simulink library "Blocks_Library"  (R2022b)
settings: Solver=VariableStepAuto  StartTime=0.0  StopTime=10.0  RelTol=1e-3
undefined symbols (not defined in the file): dataName, enumName, enumValue, raptor_xcp_function
libraries: Raptor_lib x13, $bdroot x2, simulink x1, simulink_extras x1
settings Model: Creator=jackh  LastModifiedBy=jackh

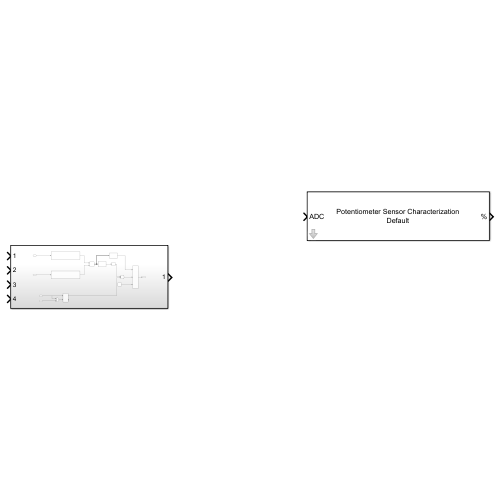
[thumbnail: Simulink's stored preview of the top-level diagram]
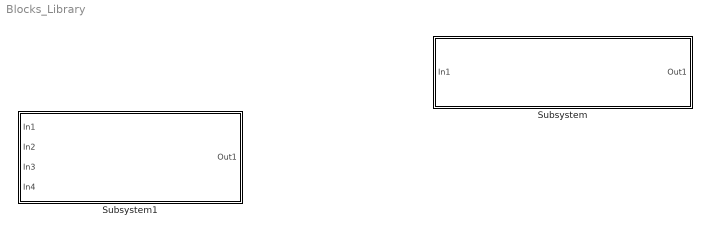
== system Blocks_Library ==
  Subsystem : Subsystem  mask{nam=Default}
      mask prompts: nam "Name"
      mask Display:
      | n = get_param(gcb, 'nam');
      | disp(['Potentiometer Sensor Characterization\n' n]);
      | port_label('input', 1, 'ADC');
      | port_label('output', 1, '%');
  Subsystem1 : Subsystem

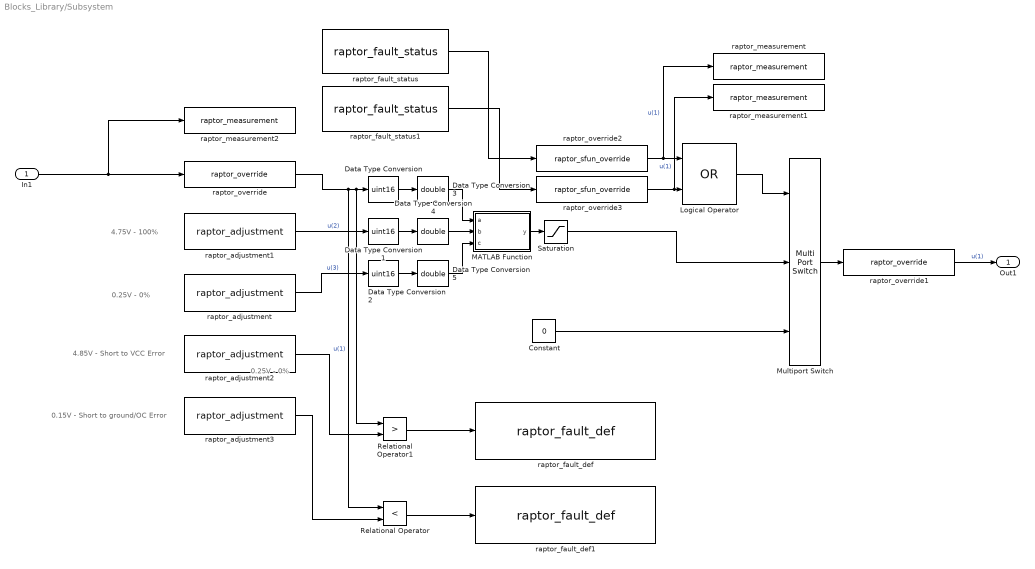
== system Blocks_Library/Subsystem ==
  note: 0.25V - 0%
  note: 4.75V - 100%
  note: 0.25V - 0%
  note: 4.85V - Short to VCC Error
  note: 0.15V - Short to ground/OC Error
  In1 : Inport
  Constant : Constant  Value=0
  Data Type Conversion : DataTypeConversion  OutDataTypeStr=uint16  SaturateOnIntegerOverflow=off  RndMeth=Floor
  Data Type Conversion1 : DataTypeConversion  OutDataTypeStr=uint16  SaturateOnIntegerOverflow=off  RndMeth=Floor
  Data Type Conversion2 : DataTypeConversion  OutDataTypeStr=uint16  SaturateOnIntegerOverflow=off  RndMeth=Floor
  Data Type Conversion3 : DataTypeConversion  OutDataTypeStr=double  SaturateOnIntegerOverflow=off  RndMeth=Floor
  Data Type Conversion4 : DataTypeConversion  OutDataTypeStr=double  SaturateOnIntegerOverflow=off  RndMeth=Floor
  Data Type Conversion5 : DataTypeConversion  OutDataTypeStr=double  SaturateOnIntegerOverflow=off  RndMeth=Floor
  Logical Operator : Logic  Operator=OR  IconShape=distinctive  AllPortsSameDT=off  OutDataTypeStr=boolean
  MATLAB Function : MATLAB Function  TreatAsAtomicUnit=on
  Multiport Switch : MultiPortSwitch  DataPortOrder=Zero-based contiguous  Inputs=2  zeroidx=on  SaturateOnIntegerOverflow=off  InputSameDT=off
  Relational Operator : RelationalOperator  Operator=<  OutDataTypeStr=boolean  RndMeth=Simplest  InputSameDT=off
  Relational Operator1 : RelationalOperator  Operator=>  OutDataTypeStr=boolean  RndMeth=Simplest  InputSameDT=off
  Saturation : Saturate  UpperLimit=100  LowerLimit=0
  raptor_adjustment : Raptor_lib/Data Storage/raptor_adjustment  paramName=[nam '_ADCLoPT']  nameSource=Parameter  initValue=205  dataType=double  storage=Constant (FLASH)  calDispType=Number  calEnum={'False', 'True'}  calGain=1.0  calOffset=0.0  calMax=inf  calMin=-inf  calFormat='-1'  calUnit='ADC'  calHelp="\"ADC Low Point\""  calAccess=1  calFunction=raptor_xcp_function(gcb)  calDispHeaders=off  calColHeaders={'Col1' 'Col2' 'Col3'}  calRowHeaders={'Row1' 'Row2' 'Row3'}
      settings: SourceProductName=Raptor
  raptor_adjustment1 : Raptor_lib/Data Storage/raptor_adjustment  paramName=[nam '_ADCHiPT']  nameSource=Parameter  initValue=3890  dataType=double  storage=Constant (FLASH)  calDispType=Number  calEnum={'False', 'True'}  calGain=1.0  calOffset=0.0  calMax=inf  calMin=-inf  calFormat='-1'  calUnit='ADC'  calHelp="\"ADC High Point\""  calAccess=1  calFunction=raptor_xcp_function(gcb)  calDispHeaders=off  calColHeaders={'Col1' 'Col2' 'Col3'}  calRowHeaders={'Row1' 'Row2' 'Row3'}
      settings: SourceProductName=Raptor
  raptor_adjustment2 : Raptor_lib/Data Storage/raptor_adjustment  paramName=[nam '_InputHighThresh']  nameSource=Parameter  initValue=3972  dataType=double  storage=Constant (FLASH)  calDispType=Number  calEnum={'False', 'True'}  calGain=1.0  calOffset=0.0  calMax=inf  calMin=-inf  calFormat='-1'  calUnit='ADC'  calHelp="\"Input out of range high point threshold\""  calAccess=1  calFunction=raptor_xcp_function(gcb)  calDispHeaders=off  calColHeaders={'Col1' 'Col2' 'Col3'}  calRowHeaders={'Row1' 'Row2' 'Row3'}
      settings: SourceProductName=Raptor
  raptor_adjustment3 : Raptor_lib/Data Storage/raptor_adjustment  paramName=[nam '_InputLowThresh']  nameSource=Parameter  initValue=123  dataType=double  storage=Constant (FLASH)  calDispType=Number  calEnum={'False', 'True'}  calGain=1.0  calOffset=0.0  calMax=inf  calMin=-inf  calFormat='-1'  calUnit='ADC'  calHelp="\"Input out of range low point threshold\""  calAccess=1  calFunction=raptor_xcp_function(gcb)  calDispHeaders=off  calColHeaders={'Col1' 'Col2' 'Col3'}  calRowHeaders={'Row1' 'Row2' 'Row3'}
      settings: SourceProductName=Raptor
  raptor_fault_def : Raptor_lib/Faults/raptor_fault_def  faultName=[nam '_InputHi']  persist=off  sticky=off  emisRelated=off  singleTrip=off  clearMethod=Standard  xLimit=25  yLimit=50  calEnable=on  addDisable=off  calAccess=4  calFunction='System | FaultManager'
      settings: SourceProductName=Raptor
  raptor_fault_def1 : Raptor_lib/Faults/raptor_fault_def  faultName=[nam '_InputLow']  persist=off  sticky=off  emisRelated=off  singleTrip=off  clearMethod=Standard  xLimit=25  yLimit=50  calEnable=on  addDisable=off  calAccess=4  calFunction='System | FaultManager'
      settings: SourceProductName=Raptor
  raptor_fault_status : Raptor_lib/Faults/raptor_fault_status  faultSource=Parameter  faultName=[nam '_InputHi']  notOccurred=off  suspected=off  active=on  occurred=off  failedThisDC=off  testCmpltThisDC=off  failing=off  pending=on  confirmed=on  mil=on  permanent=off  ready=on  prevConfirmed=off  failedSinceClear=off  failedLastDC=off  prevMil=off
      settings: SourceProductName=Raptor
  raptor_fault_status1 : Raptor_lib/Faults/raptor_fault_status  faultSource=Parameter  faultName=[nam '_InputLow']  notOccurred=off  suspected=off  active=on  occurred=off  failedThisDC=off  testCmpltThisDC=off  failing=off  pending=on  confirmed=on  mil=on  permanent=off  ready=on  prevConfirmed=off  failedSinceClear=off  failedLastDC=off  prevMil=off
      settings: SourceProductName=Raptor
  raptor_measurement : Raptor_lib/Data Storage/raptor_measurement  paramName=[nam 'HighProbe']  nameSource=Parameter  calDispType=Number  calEnum={'False', 'True'}  calGain=1.0  calOffset=0.0  calMax=inf  calMin=-inf  calFormat='-1'  calUnit=''  calHelp=''  calAccess=1  calFunction=raptor_xcp_function(gcb)  calVisible=on
      settings: SourceProductName=Raptor
  raptor_measurement1 : Raptor_lib/Data Storage/raptor_measurement  paramName=[nam 'LowProbe']  nameSource=Parameter  calDispType=Number  calEnum={'False', 'True'}  calGain=1.0  calOffset=0.0  calMax=inf  calMin=-inf  calFormat='-1'  calUnit=''  calHelp=''  calAccess=1  calFunction=raptor_xcp_function(gcb)  calVisible=on
      settings: SourceProductName=Raptor
  raptor_measurement2 : Raptor_lib/Data Storage/raptor_measurement  paramName=[nam '_ADC_Raw']  nameSource=Parameter  calDispType=Number  calEnum={'False', 'True'}  calGain=1.0  calOffset=0.0  calMax=inf  calMin=-inf  calFormat='-1'  calUnit=''  calHelp=''  calAccess=1  calFunction=raptor_xcp_function(gcb)  calVisible=on
      settings: SourceProductName=Raptor
  raptor_override : Raptor_lib/Data Storage/raptor_override  paramName=[nam '_ADC']  nameSource=Parameter  measurement=Output  calDispType=Number  calEnum={'False', 'True'}  calGain=1.0  calOffset=0.0  calMax=inf  calMin=-inf  calFormat='-1'  calUnit=''  calHelp=''  calAccess=1  calFunction="[raptor_xcp_function(gcb) '|'  'Override']"
      settings: SourceProductName=Raptor
  raptor_override1 : Raptor_lib/Data Storage/raptor_override  paramName=nam  nameSource=Parameter  measurement=Output  calDispType=Number  calEnum={'False', 'True'}  calGain=1.0  calOffset=0.0  calMax=inf  calMin=-inf  calFormat='-1'  calUnit=''  calHelp=''  calAccess=1  calFunction="[raptor_xcp_function(gcb) '|'  'Override']"
      settings: SourceProductName=Raptor
  raptor_override2 : S-Function  FunctionName=raptor_sfun_override  Parameters=char({dataName,''}), uint8(calDispType), char(enumName), int32(enumValue), double(calGain), double(calOffset), double(calMax), double(calMin), char(calUnit), char(calHelp), char(calFormat), char(calFunction), char(calAccess), uint8(measurement)  SFunctionDeploymentMode=off  EnableBusSupport=off  mask(Override){paramName=[nam '_InputHi_Override'], nameSource=Parameter, measurement=Output, calDispType=Number, calEnum={'False', 'True'}, calGain=1.0, calOffset=0.0, calMax=inf, calMin=-inf, calFormat='-1', calUnit='', calHelp='', calAccess=1, calFunction=[raptor_xcp_function(gcb) '|'  'Override']}
      mask prompts: paramName "Name:"; nameSource "Name Source:"; measurement "Add Measurement to:"; calDispType "Display as:"; calEnum "Enumeration Definition:"; calGain "Gain:"; calOffset "Offset:"; calMax "Max:"; calMin "Min:"; calFormat "Display Decimal Format:"; calUnit "Unit Text:"; calHelp "Help Text:"; calAccess "Access Level"; calFunction "Function"
      mask help: This block is used to modify the value on a wire as needed from the calibration tool.
      mask init:
      | raptor_sfun_override_maskInit;
      settings: MoveFcn=raptor_icon_redraw(gcb);
      mask Help: eval('raptor_help(''raptor_override'');')
      mask TypeOptions nameSource: Parameter | Input Wire | Output Wire
      mask Callback nameSource: raptor_sfun_override_dlgCb(gcb, 'nameSource');
      mask TypeOptions measurement: None | Input | Output
      mask TypeOptions calDispType: Number | Enumeration | String
      mask Callback calDispType: raptor_sfun_override_dlgCb(gcb, 'calDispType');
      mask TypeOptions calAccess: 4 | 3 | 2 | 1
      mask Display: raptor_sfun_override_icon;
  raptor_override3 : S-Function  FunctionName=raptor_sfun_override  Parameters=char({dataName,''}), uint8(calDispType), char(enumName), int32(enumValue), double(calGain), double(calOffset), double(calMax), double(calMin), char(calUnit), char(calHelp), char(calFormat), char(calFunction), char(calAccess), uint8(measurement)  SFunctionDeploymentMode=off  EnableBusSupport=off  mask(Override){paramName=[nam '_InputLow_Override'], nameSource=Parameter, measurement=Output, calDispType=Number, calEnum={'False', 'True'}, calGain=1.0, calOffset=0.0, calMax=inf, calMin=-inf, calFormat='-1', calUnit='', calHelp='', calAccess=1, calFunction=[raptor_xcp_function(gcb) '|'  'Override']}
      mask prompts: paramName "Name:"; nameSource "Name Source:"; measurement "Add Measurement to:"; calDispType "Display as:"; calEnum "Enumeration Definition:"; calGain "Gain:"; calOffset "Offset:"; calMax "Max:"; calMin "Min:"; calFormat "Display Decimal Format:"; calUnit "Unit Text:"; calHelp "Help Text:"; calAccess "Access Level"; calFunction "Function"
      mask help: This block is used to modify the value on a wire as needed from the calibration tool.
      mask init:
      | raptor_sfun_override_maskInit;
      settings: MoveFcn=raptor_icon_redraw(gcb);
      mask Help: eval('raptor_help(''raptor_override'');')
      mask TypeOptions nameSource: Parameter | Input Wire | Output Wire
      mask Callback nameSource: raptor_sfun_override_dlgCb(gcb, 'nameSource');
      mask TypeOptions measurement: None | Input | Output
      mask TypeOptions calDispType: Number | Enumeration | String
      mask Callback calDispType: raptor_sfun_override_dlgCb(gcb, 'calDispType');
      mask TypeOptions calAccess: 4 | 3 | 2 | 1
      mask Display: raptor_sfun_override_icon;
  Out1 : Outport
  wires:
  In1/1 -> raptor_measurement2/1, raptor_override/1
  raptor_override/1 -> Relational Operator/1, Data Type Conversion/1, Relational Operator1/1  "u(1)"
  raptor_adjustment1/1 -> Data Type Conversion1/1  "u(2)"
  raptor_adjustment/1 -> Data Type Conversion2/1  "u(3)"
  Saturation/1 -> Multiport Switch/2
  Multiport Switch/1 -> raptor_override1/1
  raptor_override1/1 -> Out1/1  "u(1)"
  raptor_adjustment2/1 -> Relational Operator1/2
  raptor_adjustment3/1 -> Relational Operator/2
  Data Type Conversion/1 -> Data Type Conversion3/1
  Data Type Conversion1/1 -> Data Type Conversion4/1
  Data Type Conversion2/1 -> Data Type Conversion5/1
  Constant/1 -> Multiport Switch/3
  Data Type Conversion4/1 -> MATLAB Function/2(b)
  Data Type Conversion5/1 -> MATLAB Function/3(c)
  Data Type Conversion3/1 -> MATLAB Function/1(a)
  MATLAB Function/1(y) -> Saturation/1
  raptor_fault_status/1 -> raptor_override2/1
  raptor_fault_status1/1 -> raptor_override3/1
  Logical Operator/1 -> Multiport Switch/1
  Relational Operator1/1 -> raptor_fault_def/1
  raptor_override2/1 -> raptor_measurement/1, Logical Operator/1  "u(1)"
  raptor_override3/1 -> raptor_measurement1/1, Logical Operator/2  "u(1)"
  Relational Operator/1 -> raptor_fault_def1/1

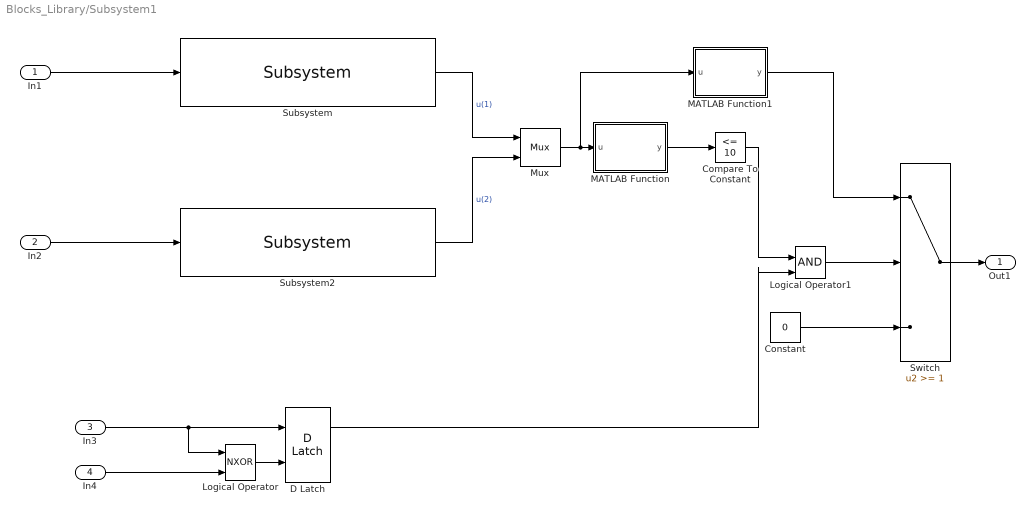
== system Blocks_Library/Subsystem1 ==
  In1 : Inport
  In2 : Inport  Port=2
  In3 : Inport  Port=3
  In4 : Inport  Port=4
  Compare To Constant : simulink/Logic and Bit Operations/Compare To Constant  relop=<=  const=10  OutDataTypeStr=uint8
  Constant : Constant  Value=0
  D Latch : simulink_extras/Flip Flops/D Latch
  Logical Operator : Logic  Operator=NXOR  IconShape=distinctive  AllPortsSameDT=off  OutDataTypeStr=boolean
  Logical Operator1 : Logic  IconShape=distinctive  AllPortsSameDT=off  OutDataTypeStr=boolean
  MATLAB Function : MATLAB Function  TreatAsAtomicUnit=on
  MATLAB Function1 : MATLAB Function  TreatAsAtomicUnit=on
  Mux : Mux  Inputs=2
      settings: DisplayOption=signals
  Subsystem : $bdroot/Subsystem  nam=POT1
  Subsystem2 : $bdroot/Subsystem  nam=POT2
  Switch : Switch  Threshold=1  SaturateOnIntegerOverflow=off  InputSameDT=off
  Out1 : Outport
  wires:
  Switch/1 -> Out1/1
  In4/1 -> Logical Operator/2
  In3/1 -> D Latch/1, Logical Operator/1
  In2/1 -> Subsystem2/1
  In1/1 -> Subsystem/1
  Mux/1 -> MATLAB Function/1(u), MATLAB Function1/1(u)
  Logical Operator1/1 -> Switch/2
  Logical Operator/1 -> D Latch/2
  Subsystem2/1 -> Mux/2  "u(2)"
  MATLAB Function/1(y) -> Compare To Constant/1
  Subsystem/1 -> Mux/1  "u(1)"
  D Latch/1 -> Logical Operator1/2
  Constant/1 -> Switch/3
  MATLAB Function1/1(y) -> Switch/1
  Compare To Constant/1 -> Logical Operator1/1

== matlab function Blocks_Library/Subsystem1/MATLAB Function ==
  data: u input; y output
function y = fcn(u)
y = abs(u(2)-u(1));
end

== matlab function Blocks_Library/Subsystem1/MATLAB Function1 ==
  data: u input; y output
function y = fcn(u)
y = (u(2)+u(1))/2;
end

== matlab function Blocks_Library/Subsystem/MATLAB Function ==
  data: a input; y output; b input; c input
function y = fcn(a,b,c)
y = ((a-c)/(b-c));
end
